simulink model "tesys"  (R2019b)
settings: Solver=VariableStepAuto  StartTime=0.0  StopTime=50  FixedStep=1e-4  MaxStep=1e-3  RelTol=1e-3  EnableMultiTasking=on
PreLoadFcn:
  | tesys_init
undefined symbols (not defined in the file or in its folder): Ts_save
libraries: simulink x2
settings Model: Creator=ricker  LastModifiedBy=isud
settings SolverCC: AlgebraicLoopSolver=LineSearch
settings DataIOCC: Decimation=10  SaveFormat=Array  SignalLoggingSaveFormat=ModelDataLogs  ReturnWorkspaceOutputs=off  OutputSaveName=yout, yout2  SignalLoggingName=sigsOut
settings OptimizationCC: LifeSpan=inf
settings DebuggingCC: SaveWithParameterizedLinksMsg=none  UnderspecifiedInitializationDetection=Classic  MergeDetectMultiDrivingBlocksExec=none  SignalResolutionControl=TryResolveAllWithWarning  MultiTaskDSMMsg=warning  MultiTaskCondExecSysMsg=none  SFUnexpectedBacktrackingDiag=warning  SFNoUnconditionalDefaultTransitionDiag=warning  SFExecutionAtInitializationDiag=none  ArithmeticOperatorsInVariantConditions=warning
settings HardwareCC: ProdBitPerPointer=32  ProdBitPerSizeT=32  ProdBitPerPtrDiffT=32  ProdLargestAtomicFloat=None  ProdIntDivRoundTo=Undefined  ProdEndianess=Unspecified  ProdWordSize=32  ProdHWDeviceType=32-bit Generic  TargetUnknown=on
settings ModelReferenceCC: PropagateSignalLabelsOutOfModel=off
settings SFSimCC: SimUseLocalCustomCode=off  CustomCodeUndefinedFunction=UseInterfaceOnly
settings RTWCC: RTWUseLocalCustomCode=off
settings CodeAppCC: StateflowObjectComments=on
settings GRTTargetCC: TargetLangStandard=C89/C90 (ANSI)  GeneratePreprocessorConditionals=Disable all  CombineOutputUpdateFcns=off  GRTInterface=on
settings ConfigComp: CovMetricSettings=dw  CovHtmlReporting=on  CovSaveCumulativeToWorkspaceVar=on  CovSaveSingleToWorkspaceVar=on  CovExternalEMLEnable=off  CovSFcnEnable=off

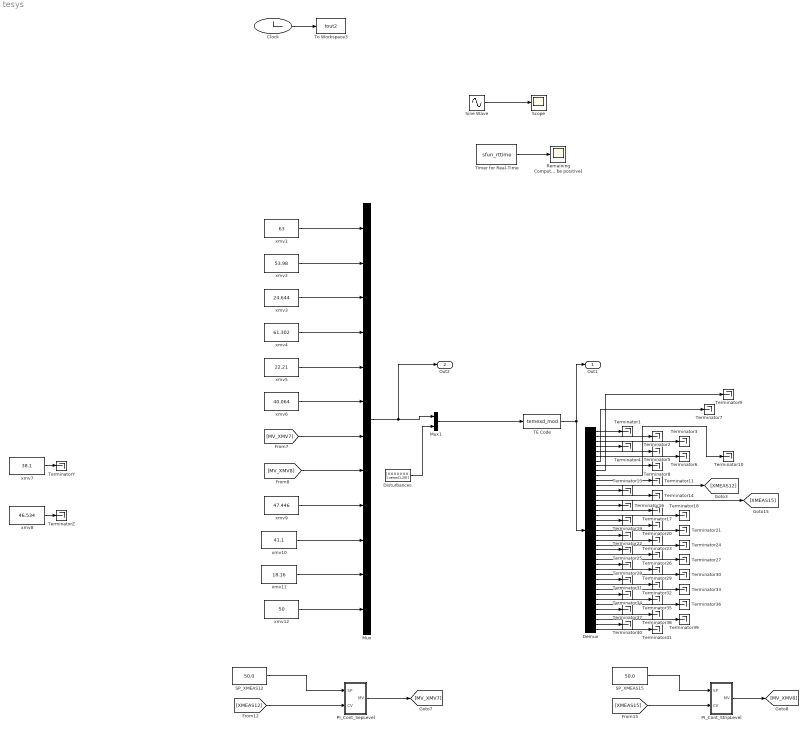
== system tesys ==
  Clock : Clock
  Demux : Demux  Outputs=41
  Disturbances : Constant  Value=[ 0 0 0 0 0 0 0 1 zeros(1,20)]
  Mux : Mux  Inputs=12
  Mux1 : Mux  Inputs=2
  PI_Cont_SepLevel : Subsystem  mask{P_Gain=2, I_Gain=0.1, V_Bias=38.1, V_Low=0, V_High=100}
      mask prompts: P_Gain "P"; I_Gain "I"; V_Bias "Valve Opening (Bias)"; V_Low "Valve Opening (Low)"; V_High "Valve Opening (High)"
      mask DialogControl Container5 Prompt: Controller Parameters
      mask DialogControl ParameterGroupVar Prompt: Valve Parameters
  PI_Cont_StripLevel : Subsystem  mask{P_Gain=2, I_Gain=0.1, V_Bias=46.5, V_Low=0, V_High=100}
      mask prompts: P_Gain "P"; I_Gain "I"; V_Bias "Valve Opening (Bias)"; V_Low "Valve Opening (Low)"; V_High "Valve Opening (High)"
      mask DialogControl Container5 Prompt: Controller Parameters
      mask DialogControl ParameterGroupVar Prompt: Valve Parameters
  Remaining Computation Time (must be positive) : Scope
  SP_XMEAS12 : Constant  Value=50.0  OutDataTypeStr=double
  SP_XMEAS15 : Constant  Value=50.0  OutDataTypeStr=double
  Scope : Scope
  Sine Wave : Sin  SampleTime=0
  TE Code : S-Function  FunctionName=temexd_mod  Parameters=[], [], 0  SFunctionDeploymentMode=off  EnableBusSupport=off
  Terminator{1..11,13..14,16..41} (39 alike) : Terminator
  TerminatorY : Terminator
  TerminatorZ : Terminator
  Timer for Real-Time : S-Function  FunctionName=sfun_rttime  Parameters=100  SFunctionDeploymentMode=off  EnableBusSupport=off
  To Workspace3 : ToWorkspace  VariableName=tout2  SampleTime=Ts_save
  xmv1 : Constant  Value=63
  xmv10 : Constant  Value=41.1
  xmv11 : Constant  Value=18.16
  xmv12 : Constant  Value=50
  xmv2 : Constant  Value=53.98
  xmv3 : Constant  Value=24.644
  xmv4 : Constant  Value=61.302
  xmv5 : Constant  Value=22.21
  xmv6 : Constant  Value=40.064
  xmv7 : Constant  Value=38.1
  xmv8 : Constant  Value=46.534
  xmv9 : Constant  Value=47.446
  Out1 : Outport
  Out2 : Outport  Port=2
  wires:
  Mux1/1 -> TE Code/1
  TE Code/1 -> Demux/1, Out1/1
  Timer for Real-Time/1 -> Remaining Computation Time (must be positive)/1
  Sine Wave/1 -> Scope/1
  xmv1/1 -> Mux/1
  xmv2/1 -> Mux/2
  xmv3/1 -> Mux/3
  xmv4/1 -> Mux/4
  xmv5/1 -> Mux/5
  xmv6/1 -> Mux/6
  [MV_XMV7] -> Mux/7
  xmv9/1 -> Mux/9
  xmv10/1 -> Mux/10
  xmv11/1 -> Mux/11
  xmv12/1 -> Mux/12
  Disturbances/1 -> Mux1/2
  Mux/1 -> Out2/1, Mux1/1
  Clock/1 -> To Workspace3/1
  Demux/1 -> Terminator1/1
  Demux/2 -> Terminator2/1
  Demux/3 -> Terminator3/1
  Demux/4 -> Terminator4/1
  Demux/6 -> Terminator6/1
  Demux/5 -> Terminator5/1
  Demux/7 -> Terminator7/1
  Demux/8 -> Terminator8/1
  Demux/9 -> Terminator9/1
  Demux/11 -> Terminator11/1
  Demux/10 -> Terminator10/1
  Demux/13 -> Terminator13/1
  Demux/14 -> Terminator14/1
  Demux/15 -> [XMEAS15]
  Demux/16 -> Terminator16/1
  Demux/17 -> Terminator17/1
  Demux/18 -> Terminator18/1
  Demux/19 -> Terminator19/1
  Demux/20 -> Terminator20/1
  Demux/21 -> Terminator21/1
  Demux/22 -> Terminator22/1
  Demux/23 -> Terminator23/1
  Demux/24 -> Terminator24/1
  Demux/25 -> Terminator25/1
  Demux/26 -> Terminator26/1
  Demux/27 -> Terminator27/1
  Demux/28 -> Terminator28/1
  Demux/29 -> Terminator29/1
  Demux/30 -> Terminator30/1
  Demux/31 -> Terminator31/1
  Demux/32 -> Terminator32/1
  Demux/33 -> Terminator33/1
  Demux/34 -> Terminator34/1
  Demux/35 -> Terminator35/1
  Demux/36 -> Terminator36/1
  Demux/37 -> Terminator37/1
  Demux/38 -> Terminator38/1
  Demux/39 -> Terminator39/1
  Demux/40 -> Terminator40/1
  Demux/41 -> Terminator41/1
  SP_XMEAS12/1 -> PI_Cont_SepLevel/1(SP)
  [XMEAS12] -> PI_Cont_SepLevel/2(CV)
  PI_Cont_SepLevel/1(MV) -> [MV_XMV7]
  xmv7/1 -> TerminatorY/1
  SP_XMEAS15/1 -> PI_Cont_StripLevel/1(SP)
  [XMEAS15] -> PI_Cont_StripLevel/2(CV)
  PI_Cont_StripLevel/1(MV) -> [MV_XMV8]
  [MV_XMV8] -> Mux/8
  xmv8/1 -> TerminatorZ/1
  Demux/12 -> [XMEAS12]

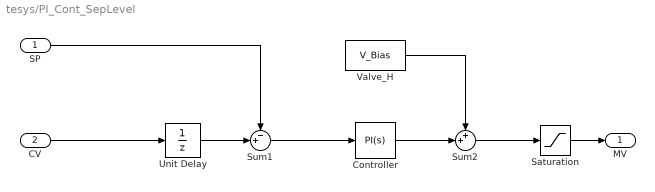
== system tesys/PI_Cont_SepLevel ==
  SP : Inport
  CV : Inport  Port=2
  Controller : simulink/Continuous/PID Controller  Controller=PI  Form=Parallel  TimeDomain=Continuous-time  SampleTime=-1  IntegratorMethod=Forward Euler  FilterMethod=Forward Euler  ControllerParametersSource=internal  P=P_Gain  I=I_Gain  D=0  UseFilter=on  N=100  TunerSelectOption=Transfer Function Based (PID Tuner App)  InitialConditionSource=internal  InitialConditionForIntegrator=0  InitialConditionForFilter=0  DifferentiatorICPrevScaledInput=0  ExternalReset=none  TrackingMode=off  Kt=1  LimitOutput=off  UpperSaturationLimit=inf  LowerSaturationLimit=-inf  LinearizeAsGain=on  AntiWindupMode=none  Kb=1  POutMin=[]  POutMax=[]  IOutMin=[]  IOutMax=[]  DOutMin=[]  DOutMax=[]  NOutMin=[]  NOutMax=[]  SumOutMin=[]  SumOutMax=[]  SaturationOutMin=[]  SaturationOutMax=[]  PParamMin=[]  PParamMax=[]  IParamMin=[]  IParamMax=[]  DParamMin=[]  DParamMax=[]  NParamMin=[]  NParamMax=[]  KbParamMin=[]  KbParamMax=[]  KtParamMin=[]  KtParamMax=[]  KbOutMin=[]  KbOutMax=[]  KtOutMin=[]  KtOutMax=[]  IntegratorOutMin=[]  IntegratorOutMax=[]  FilterOutMin=[]  FilterOutMax=[]  SumI1OutMin=[]  SumI1OutMax=[]  SumI2OutMin=[]  SumI2OutMax=[]  SumI3OutMin=[]  SumI3OutMax=[]  SumI4OutMin=[]  SumI4OutMax=[]  SumDOutMin=[]  SumDOutMax=[]  DifferentiatorOutMin=[]  DifferentiatorOutMax=[]  FilterDiffOutCoefMin=[]  FilterDiffOutCoefMax=[]  ReciprocalOutMin=[]  ReciprocalOutMax=[]  SumDenOutMin=[]  SumDenOutMax=[]  SumNumOutMin=[]  SumNumOutMax=[]  DivideOutMin=[]  DivideOutMax=[]  IntegratorContinuousStateAttributes=''  IntegratorStateMustResolveToSignalObject=off  IntegratorRTWStateStorageClass=Auto  FilterContinuousStateAttributes=''  FilterStateMustResolveToSignalObject=off  FilterRTWStateStorageClass=Auto  ParallelPVariant=InternalParameters  IdealPVariant=Disabled  IVariant=InternalParameters  DVariant=Disabled  IntegratorVariant=Continuous  SatVariant=Disabled  AWVariant=Passthrough  PCopyVariant=Disabled  TRVariant=Disabled  FdbkBlocksVariant=Forward  IdealPFdbkVariant=Disabled  SatFdbkVariant=Disabled  DerivativeFilterVariant=Disabled  NVariant=Disabled  NCopyVariant=Disabled_SignalSpec  FilterICVariant=Disabled  IntegratorICVariant=InternalICs  ExternalResetVariant=Disabled  TRSumVariant=Passthrough  SumFdbkVariant=Disabled  SumVariant=Sum_PI
  Saturation : Saturate  UpperLimit=V_High  LowerLimit=V_Low
  Sum1 : Sum  Inputs=-+|  OutDataTypeStr=double  InputSameDT=on
  Sum2 : Sum  Inputs=++|  OutDataTypeStr=double
  Unit Delay : UnitDelay  InitialCondition=45  SampleTime=-1  HasFrameUpgradeWarning=on
  Valve_H : Constant  Value=V_Bias
  MV : Outport
  wires:
  SP/1 -> Sum1/1
  Sum2/1 -> Saturation/1
  CV/1 -> Unit Delay/1
  Sum1/1 -> Controller/1
  Controller/1 -> Sum2/2
  Unit Delay/1 -> Sum1/2
  Valve_H/1 -> Sum2/1
  Saturation/1 -> MV/1

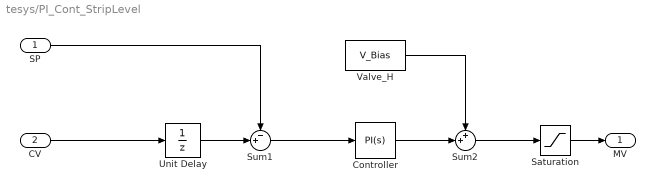
== system tesys/PI_Cont_StripLevel ==
  SP : Inport
  CV : Inport  Port=2
  Controller : simulink/Continuous/PID Controller  Controller=PI  Form=Parallel  TimeDomain=Continuous-time  SampleTime=-1  IntegratorMethod=Forward Euler  FilterMethod=Forward Euler  ControllerParametersSource=internal  P=P_Gain  I=I_Gain  D=0  UseFilter=on  N=100  TunerSelectOption=Transfer Function Based (PID Tuner App)  InitialConditionSource=internal  InitialConditionForIntegrator=0  InitialConditionForFilter=0  DifferentiatorICPrevScaledInput=0  ExternalReset=none  TrackingMode=off  Kt=1  LimitOutput=off  UpperSaturationLimit=inf  LowerSaturationLimit=-inf  LinearizeAsGain=on  AntiWindupMode=none  Kb=1  POutMin=[]  POutMax=[]  IOutMin=[]  IOutMax=[]  DOutMin=[]  DOutMax=[]  NOutMin=[]  NOutMax=[]  SumOutMin=[]  SumOutMax=[]  SaturationOutMin=[]  SaturationOutMax=[]  PParamMin=[]  PParamMax=[]  IParamMin=[]  IParamMax=[]  DParamMin=[]  DParamMax=[]  NParamMin=[]  NParamMax=[]  KbParamMin=[]  KbParamMax=[]  KtParamMin=[]  KtParamMax=[]  KbOutMin=[]  KbOutMax=[]  KtOutMin=[]  KtOutMax=[]  IntegratorOutMin=[]  IntegratorOutMax=[]  FilterOutMin=[]  FilterOutMax=[]  SumI1OutMin=[]  SumI1OutMax=[]  SumI2OutMin=[]  SumI2OutMax=[]  SumI3OutMin=[]  SumI3OutMax=[]  SumI4OutMin=[]  SumI4OutMax=[]  SumDOutMin=[]  SumDOutMax=[]  DifferentiatorOutMin=[]  DifferentiatorOutMax=[]  FilterDiffOutCoefMin=[]  FilterDiffOutCoefMax=[]  ReciprocalOutMin=[]  ReciprocalOutMax=[]  SumDenOutMin=[]  SumDenOutMax=[]  SumNumOutMin=[]  SumNumOutMax=[]  DivideOutMin=[]  DivideOutMax=[]  IntegratorContinuousStateAttributes=''  IntegratorStateMustResolveToSignalObject=off  IntegratorRTWStateStorageClass=Auto  FilterContinuousStateAttributes=''  FilterStateMustResolveToSignalObject=off  FilterRTWStateStorageClass=Auto  ParallelPVariant=InternalParameters  IdealPVariant=Disabled  IVariant=InternalParameters  DVariant=Disabled  IntegratorVariant=Continuous  SatVariant=Disabled  AWVariant=Passthrough  PCopyVariant=Disabled  TRVariant=Disabled  FdbkBlocksVariant=Forward  IdealPFdbkVariant=Disabled  SatFdbkVariant=Disabled  DerivativeFilterVariant=Disabled  NVariant=Disabled  NCopyVariant=Disabled_SignalSpec  FilterICVariant=Disabled  IntegratorICVariant=InternalICs  ExternalResetVariant=Disabled  TRSumVariant=Passthrough  SumFdbkVariant=Disabled  SumVariant=Sum_PI
  Saturation : Saturate  UpperLimit=V_High  LowerLimit=V_Low
  Sum1 : Sum  Inputs=-+|  OutDataTypeStr=double  InputSameDT=on
  Sum2 : Sum  Inputs=++|  OutDataTypeStr=double
  Unit Delay : UnitDelay  InitialCondition=45  SampleTime=-1  HasFrameUpgradeWarning=on
  Valve_H : Constant  Value=V_Bias
  MV : Outport
  wires:
  SP/1 -> Sum1/1
  Sum2/1 -> Saturation/1
  CV/1 -> Unit Delay/1
  Sum1/1 -> Controller/1
  Controller/1 -> Sum2/2
  Unit Delay/1 -> Sum1/2
  Valve_H/1 -> Sum2/1
  Saturation/1 -> MV/1
